simulink library "CommercialVehicleLibrary2G"  (R2021a)
settings: Solver=VariableStepAuto  StartTime=0.0  StopTime=10.0  RelTol=1e-3
values from neighbouring files (symbols this model uses):
  brake_input = [0   tmax ... (first row only)    [init_vehicle.m]    (also in run_Circle.m = [0  tmax; run_Coastdown.m = [0  2  tmax; run_DoubleLaneChangeDriver.m = [0   2  tmax; run_MaxAcc.m = [0  2  tmax)
  pose_t0 = [0 0 0 0]    [init_vehicle.m]    (also in run_Circle.m; run_Coastdown.m; run_DoubleLaneChangeDriver.m; run_MaxAcc.m)
  rdfname = 'TNO_FlatRoad.rdf'    [run_Circle.m]    (also in run_Coastdown.m; run_DoubleLaneChangeDriver.m; run_MaxAcc.m; run_Rollover.m)
  rdfname_inner = 'TNO_FlatRoad.rdf'    [run_Circle.m]    (also in run_Coastdown.m; run_DoubleLaneChangeDriver.m; run_MaxAcc.m; run_Rollover.m)
  steer_input = [0  tmax ... (first row only)    [init_vehicle.m]    (also in run_Circle.m = [0  2   10     13       tmax; run_Coastdown.m = [0 tmax; run_DoubleLaneChangeDriver.m = [0 tmax; run_MaxAcc.m = [0 tmax)
  throttle_input = [0         tmax ... (first row only)    [init_vehicle.m]    (also in run_Circle.m; run_Coastdown.m = [0        10         10.0001 tmax; run_DoubleLaneChangeDriver.m = [0        tmax; run_MaxAcc.m = [0        tmax)
  Vx = 0    [init_vehicle.m]    (also in run_Circle.m = Vx_kmh/3.6; run_Coastdown.m = Vx_kmh/3.6; run_DoubleLaneChangeDriver.m = Vx_kmh/3.6; run_MaxAcc.m)
  Vx_input = [0  tmax ... (first row only)    [init_vehicle.m]    (also in run_Circle.m; run_Coastdown.m = [0 tmax; run_DoubleLaneChangeDriver.m = [0 tmax; run_MaxAcc.m = [0 tmax)
undefined symbols (not defined in the file or in its folder): Drive, Floor, Fzstat, Fzstat1, Fzstat3, l, l_load1, l_load2, lbar, mass_load1, mass_load2, psi_semitrailer, rho, rim_Ixx, rim_Iyy, rim_mass, Steer, steer_path, tpfname, X, x_torsion, xcg, xcg1, xcg2, xcg_front, xcg_rear, xdrive1, xload1, xload2, xpos1, xref, xrev1, Xt0, Y, Yt0, Z
libraries: sm_lib x291, $bdroot x157, nesl_utility x143, vrlib x1
(part 12 of 12)

== system CommercialVehicleLibrary2G/Vehicles/Rigid Truck - 4 axles/Measurements ==
  Bus Creator2 : BusCreator  Inputs=3
  Bus Creator3 : BusCreator  Inputs=3
  Fcn4 : Fcn  Expr=u(3)
  PS-Simulink Converter{3..8,10..11} (8 alike) : nesl_utility/PS-Simulink Converter  PhysicalDomain=network_engine_domain  SubClassName=ps_output  LeftPortType=input  RightPortType=output  PseudoPeriodic=off  Frequencies=[]  Unit=inherit  AffineConversion=off
  Scope : Scope
  Scope1 : Scope
  Transform Sensor1 : sm_lib/Frames and Transforms/Transform Sensor  MeasurementFrame=NonRotatingFollower  SenseAngle=off  SenseAxis=off  SenseAngle1=off  SenseAngle2=off  SenseAngle3=off  SenseQ=off  SenseR=off  SenseOmegaX=on  SenseOmegaY=on  SenseOmegaZ=on  SenseOmega1=off  SenseOmega2=off  SenseOmega3=off  SenseQDot=off  SenseRDot=off  SenseAlphaX=on  SenseAlphaY=on  SenseAlphaZ=on  SenseAlpha1=off  SenseAlpha2=off  SenseAlpha3=off  SenseQDDot=off  SenseRDDot=off  SenseX=off  SenseY=off  SenseZ=off  SenseRad=off  SenseAzim=off  SenseDist=off  SenseInc=off  SenseXDot=on  SenseYDot=on  SenseZDot=off  SenseRadDot=off  SenseAzimDot=off  SenseDistDot=off  SenseIncDot=off  SenseXDDot=off  SenseYDDot=off  SenseZDDot=off  SenseRadDDot=off  SenseAzimDDot=off  SenseDistDDot=off  SenseIncDDot=off
  Transform Sensor2 : PMIOPort  Side=Left
  Transform Sensor3 : PMIOPort  Port=2  Side=Right
  Out1 : Outport
  Out2 : Outport  Port=2
  Out3 : Outport  Port=3
  wires:
  PS-Simulink Converter3/1 -> Bus Creator2/3
  PS-Simulink Converter5/1 -> Bus Creator2/1
  PS-Simulink Converter10/1 -> Scope1/1
  PS-Simulink Converter7/1 -> Bus Creator3/2
  Bus Creator2/1 -> Fcn4/1
  PS-Simulink Converter8/1 -> Bus Creator3/1
  Bus Creator3/1 -> Out2/1
  PS-Simulink Converter6/1 -> Bus Creator3/3
  PS-Simulink Converter4/1 -> Bus Creator2/2
  Fcn4/1 -> Out1/1
  PS-Simulink Converter11/1 -> Out3/1, Scope/1
  connections:
  PS-Simulink Converter11/LConn1 -- Transform Sensor1/RConn8
  PS-Simulink Converter7/LConn1 -- Transform Sensor1/RConn6
  Transform Sensor1/RConn2 -- PS-Simulink Converter5/LConn1
  PS-Simulink Converter6/LConn1 -- Transform Sensor1/RConn7
  PS-Simulink Converter3/LConn1 -- Transform Sensor1/RConn4
  Transform Sensor1/RConn1 -- Transform Sensor3/RConn1
  PS-Simulink Converter8/LConn1 -- Transform Sensor1/RConn5
  PS-Simulink Converter4/LConn1 -- Transform Sensor1/RConn3
  Transform Sensor1/RConn9 -- PS-Simulink Converter10/LConn1
  Transform Sensor1/LConn1 -- Transform Sensor2/RConn1

== system CommercialVehicleLibrary2G/Vehicles/Tractor/Cameras ==
  Front Camera Transform : sm_lib/Frames and Transforms/Rigid Transform  TranslationMethod=Cartesian  TranslationStandardOffset=0  TranslationLengthUnit=m  TranslationStandardAxis=+Z  TranslationCartesianOffset=[-10 0 6]  TranslationROffset=0  TranslationROffsetUnits=m  TranslationZOffset=0  TranslationZOffsetUnits=m  TranslationThetaOffset=0  TranslationThetaOffsetUnits=deg  RotationMethod=None  RotationAngleUnits=deg  RotationStandardAxis=+Y  RotationAngle=90  RotationArbitraryAxis=[0 0 1]  FollAlignAxisA=+X  BaseAlignAxisA=+Y  FollAlignAxisB=+Y  BaseAlignAxisB=+Z  RotationSequenceAxes=FollowerAxes  RotationSequence=XYX  RotationSequenceAngles=[0 0 0]  RotationSequenceAnglesUnits=deg  RotationMatrix=[1 0 0; 0 1 0; 0 0 1]
  Side Camera Transform : sm_lib/Frames and Transforms/Rigid Transform  TranslationMethod=Cartesian  TranslationStandardOffset=0  TranslationLengthUnit=m  TranslationStandardAxis=+Z  TranslationCartesianOffset=[5 3 3]  TranslationROffset=0  TranslationROffsetUnits=m  TranslationZOffset=0  TranslationZOffsetUnits=m  TranslationThetaOffset=0  TranslationThetaOffsetUnits=deg  RotationMethod=None  RotationAngleUnits=deg  RotationStandardAxis=+Z  RotationAngle=90  RotationArbitraryAxis=[0 0 1]  FollAlignAxisA=+X  BaseAlignAxisA=+Y  FollAlignAxisB=+Y  BaseAlignAxisB=+Z  RotationSequenceAxes=FollowerAxes  RotationSequence=XYX  RotationSequenceAngles=[0 0 0]  RotationSequenceAnglesUnits=deg  RotationMatrix=[1 0 0; 0 1 0; 0 0 1]
  Spherical Solid : sm_lib/Body Elements/Spherical Solid  GraphicAmbientColor=[0.15 0.15 0.15 1.0]  BasedOnType=Density  CenterOfMass=[0 0 0]  CenterOfMassUnits=m  GraphicDiffuseColor=[0.5 0.5 0.5]  Density=1000  DensityUnits=kg/m^3  DoExposeReferenceFrame=on  GraphicEmissiveColor=[0.0 0.0 0.0 1.0]  ExportEntireGeometry=off  SerializedExposedGeometries=<ExposedGeometries/>  SerializedFrames=<Frames/>  MarkerShape=Sphere  MarkerSize=10  GraphicType=FromGeometry  InertiaType=PointMass  Mass=1e-09  MassUnits=kg  MomentsOfInertia=[1 1 1]  MomentsOfInertiaUnits=kg*m^2  GraphicOpacity=0  ProductsOfInertia=[0 0 0]  ProductsOfInertiaUnits=kg*m^2  GraphicShininess=75  GraphicSpecularColor=[0.5 0.5 0.5 1.0]  SphereRadius=1e-09  SphereRadiusUnits=m  GraphicVisPropType=SimpleVisualProperties
  Spherical Solid1 : sm_lib/Body Elements/Spherical Solid  GraphicAmbientColor=[0.15 0.15 0.15 1.0]  BasedOnType=Density  CenterOfMass=[0 0 0]  CenterOfMassUnits=m  GraphicDiffuseColor=[0.5 0.5 0.5]  Density=1000  DensityUnits=kg/m^3  DoExposeReferenceFrame=on  GraphicEmissiveColor=[0.0 0.0 0.0 1.0]  ExportEntireGeometry=off  SerializedExposedGeometries=<ExposedGeometries/>  SerializedFrames=<Frames/>  MarkerShape=Sphere  MarkerSize=10  GraphicType=FromGeometry  InertiaType=PointMass  Mass=1e-09  MassUnits=kg  MomentsOfInertia=[1 1 1]  MomentsOfInertiaUnits=kg*m^2  GraphicOpacity=0  ProductsOfInertia=[0 0 0]  ProductsOfInertiaUnits=kg*m^2  GraphicShininess=75  GraphicSpecularColor=[0.5 0.5 0.5 1.0]  SphereRadius=1e-09  SphereRadiusUnits=m  GraphicVisPropType=SimpleVisualProperties
  " " : PMIOPort  Side=Left
  connections:
  Spherical Solid1/RConn1 -- Front Camera Transform/RConn1
  Spherical Solid/RConn1 -- Side Camera Transform/RConn1
  " "/RConn1 -- Front Camera Transform/LConn1 -- Side Camera Transform/LConn1

== system CommercialVehicleLibrary2G/Vehicles/Tractor/Measurements ==
  Bus Creator2 : BusCreator  Inputs=3
  Bus Creator3 : BusCreator  Inputs=3
  Fcn4 : Fcn  Expr=u(3)
  PS-Simulink Converter{3..8,10..11} (8 alike) : nesl_utility/PS-Simulink Converter  PhysicalDomain=network_engine_domain  SubClassName=ps_output  LeftPortType=input  RightPortType=output  PseudoPeriodic=off  Frequencies=[]  Unit=inherit  AffineConversion=off
  Scope : Scope
  Scope1 : Scope
  Transform Sensor1 : sm_lib/Frames and Transforms/Transform Sensor  MeasurementFrame=NonRotatingFollower  SenseAngle=off  SenseAxis=off  SenseAngle1=off  SenseAngle2=off  SenseAngle3=off  SenseQ=off  SenseR=off  SenseOmegaX=on  SenseOmegaY=on  SenseOmegaZ=on  SenseOmega1=off  SenseOmega2=off  SenseOmega3=off  SenseQDot=off  SenseRDot=off  SenseAlphaX=on  SenseAlphaY=on  SenseAlphaZ=on  SenseAlpha1=off  SenseAlpha2=off  SenseAlpha3=off  SenseQDDot=off  SenseRDDot=off  SenseX=off  SenseY=off  SenseZ=off  SenseRad=off  SenseAzim=off  SenseDist=off  SenseInc=off  SenseXDot=on  SenseYDot=on  SenseZDot=off  SenseRadDot=off  SenseAzimDot=off  SenseDistDot=off  SenseIncDot=off  SenseXDDot=off  SenseYDDot=off  SenseZDDot=off  SenseRadDDot=off  SenseAzimDDot=off  SenseDistDDot=off  SenseIncDDot=off
  Transform Sensor2 : PMIOPort  Side=Left
  Transform Sensor3 : PMIOPort  Port=2  Side=Right
  Out1 : Outport
  Out2 : Outport  Port=2
  Out3 : Outport  Port=3
  wires:
  PS-Simulink Converter11/1 -> Scope/1, Out3/1
  Fcn4/1 -> Out1/1
  PS-Simulink Converter4/1 -> Bus Creator2/2
  PS-Simulink Converter6/1 -> Bus Creator3/3
  Bus Creator3/1 -> Out2/1
  PS-Simulink Converter8/1 -> Bus Creator3/1
  Bus Creator2/1 -> Fcn4/1
  PS-Simulink Converter7/1 -> Bus Creator3/2
  PS-Simulink Converter10/1 -> Scope1/1
  PS-Simulink Converter5/1 -> Bus Creator2/1
  PS-Simulink Converter3/1 -> Bus Creator2/3
  connections:
  Transform Sensor1/LConn1 -- Transform Sensor2/RConn1
  Transform Sensor1/RConn9 -- PS-Simulink Converter10/LConn1
  PS-Simulink Converter4/LConn1 -- Transform Sensor1/RConn3
  PS-Simulink Converter8/LConn1 -- Transform Sensor1/RConn5
  Transform Sensor1/RConn1 -- Transform Sensor3/RConn1
  PS-Simulink Converter3/LConn1 -- Transform Sensor1/RConn4
  PS-Simulink Converter6/LConn1 -- Transform Sensor1/RConn7
  Transform Sensor1/RConn2 -- PS-Simulink Converter5/LConn1
  PS-Simulink Converter7/LConn1 -- Transform Sensor1/RConn6
  PS-Simulink Converter11/LConn1 -- Transform Sensor1/RConn8

== system CommercialVehicleLibrary2G/Combinations/LZV_B/To_workspace_semitrailer1/Subsystem ==
  In1 : Inport
  Bus Selector24 : BusSelector  OutputSignals=axle1.Tire_L.Fx,axle1.Tire_R.Fx,axle2.Tire_L.Fx,axle2.Tire_R.Fx,axle3.Tire_L.Fx,axle3.Tire_R.Fx
  Mux : Mux  Inputs=6
  Out1 : Outport
  wires:
  Bus Selector24/4 -> Mux/4  "<Fx>"
  Bus Selector24/3 -> Mux/3  "<Fx>"
  Bus Selector24/2 -> Mux/2  "<Fx>"
  Bus Selector24/1 -> Mux/1  "<Fx>"
  Mux/1 -> Out1/1
  In1/1 -> Bus Selector24/1
  Bus Selector24/5 -> Mux/5  "<Fx>"
  Bus Selector24/6 -> Mux/6  "<Fx>"

== system CommercialVehicleLibrary2G/Combinations/LZV_B/To_workspace_semitrailer1/Subsystem1 ==
  In1 : Inport
  Bus Selector24 : BusSelector  OutputSignals=axle1.Tire_L.Fy,axle1.Tire_R.Fy,axle2.Tire_L.Fy,axle2.Tire_R.Fy,axle3.Tire_L.Fy,axle3.Tire_R.Fy
  Mux : Mux  Inputs=6
  Out1 : Outport
  wires:
  Mux/1 -> Out1/1
  In1/1 -> Bus Selector24/1
  Bus Selector24/1 -> Mux/1  "<Fy>"
  Bus Selector24/2 -> Mux/2  "<Fy>"
  Bus Selector24/3 -> Mux/3  "<Fy>"
  Bus Selector24/4 -> Mux/4  "<Fy>"
  Bus Selector24/5 -> Mux/5  "<Fy>"
  Bus Selector24/6 -> Mux/6  "<Fy>"

== system CommercialVehicleLibrary2G/Combinations/LZV_B/To_workspace_semitrailer1/Subsystem2 ==
  In1 : Inport
  Bus Selector24 : BusSelector  OutputSignals=axle1.Tire_L.Fz,axle1.Tire_R.Fz,axle2.Tire_L.Fz,axle2.Tire_R.Fz,axle3.Tire_L.Fz,axle3.Tire_R.Fz
  Mux : Mux  Inputs=6
  Out1 : Outport
  wires:
  Mux/1 -> Out1/1
  In1/1 -> Bus Selector24/1
  Bus Selector24/1 -> Mux/1  "<Fz>"
  Bus Selector24/2 -> Mux/2  "<Fz>"
  Bus Selector24/3 -> Mux/3  "<Fz>"
  Bus Selector24/4 -> Mux/4  "<Fz>"
  Bus Selector24/5 -> Mux/5  "<Fz>"
  Bus Selector24/6 -> Mux/6  "<Fz>"

== system CommercialVehicleLibrary2G/Combinations/LZV_B/To_workspace_semitrailer1/Subsystem3 ==
  In1 : Inport
  Bus Selector6 : BusSelector  OutputSignals=axle1.Omega1,axle1.Omega2,axle2.Omega1,axle2.Omega2,axle3.Omega1,axle3.Omega2
  Mux : Mux  Inputs=6
  Out1 : Outport
  wires:
  In1/1 -> Bus Selector6/1
  Mux/1 -> Out1/1
  Bus Selector6/1 -> Mux/1  "<Omega1>"
  Bus Selector6/2 -> Mux/2  "<Omega2>"
  Bus Selector6/3 -> Mux/3  "<Omega1>"
  Bus Selector6/4 -> Mux/4  "<Omega2>"
  Bus Selector6/5 -> Mux/5  "<Omega1>"
  Bus Selector6/6 -> Mux/6  "<Omega2>"

== system CommercialVehicleLibrary2G/Combinations/LZV_B/To_workspace_semitrailer2/Subsystem ==
  In1 : Inport
  Bus Selector24 : BusSelector  OutputSignals=axle1.Tire_L.Fx,axle1.Tire_R.Fx,axle2.Tire_L.Fx,axle2.Tire_R.Fx,axle3.Tire_L.Fx,axle3.Tire_R.Fx
  Mux : Mux  Inputs=6
  Out1 : Outport
  wires:
  Bus Selector24/6 -> Mux/6  "<Fx>"
  Bus Selector24/5 -> Mux/5  "<Fx>"
  In1/1 -> Bus Selector24/1
  Mux/1 -> Out1/1
  Bus Selector24/1 -> Mux/1  "<Fx>"
  Bus Selector24/2 -> Mux/2  "<Fx>"
  Bus Selector24/3 -> Mux/3  "<Fx>"
  Bus Selector24/4 -> Mux/4  "<Fx>"

== system CommercialVehicleLibrary2G/Combinations/LZV_B/To_workspace_semitrailer2/Subsystem1 ==
  In1 : Inport
  Bus Selector24 : BusSelector  OutputSignals=axle1.Tire_L.Fy,axle1.Tire_R.Fy,axle2.Tire_L.Fy,axle2.Tire_R.Fy,axle3.Tire_L.Fy,axle3.Tire_R.Fy
  Mux : Mux  Inputs=6
  Out1 : Outport
  wires:
  Bus Selector24/6 -> Mux/6  "<Fy>"
  Bus Selector24/5 -> Mux/5  "<Fy>"
  Bus Selector24/4 -> Mux/4  "<Fy>"
  Bus Selector24/3 -> Mux/3  "<Fy>"
  Bus Selector24/2 -> Mux/2  "<Fy>"
  Bus Selector24/1 -> Mux/1  "<Fy>"
  In1/1 -> Bus Selector24/1
  Mux/1 -> Out1/1

== system CommercialVehicleLibrary2G/Combinations/LZV_B/To_workspace_semitrailer2/Subsystem2 ==
  In1 : Inport
  Bus Selector24 : BusSelector  OutputSignals=axle1.Tire_L.Fz,axle1.Tire_R.Fz,axle2.Tire_L.Fz,axle2.Tire_R.Fz,axle3.Tire_L.Fz,axle3.Tire_R.Fz
  Mux : Mux  Inputs=6
  Out1 : Outport
  wires:
  Bus Selector24/6 -> Mux/6  "<Fz>"
  Bus Selector24/5 -> Mux/5  "<Fz>"
  Bus Selector24/4 -> Mux/4  "<Fz>"
  Bus Selector24/3 -> Mux/3  "<Fz>"
  Bus Selector24/2 -> Mux/2  "<Fz>"
  Bus Selector24/1 -> Mux/1  "<Fz>"
  In1/1 -> Bus Selector24/1
  Mux/1 -> Out1/1

== system CommercialVehicleLibrary2G/Combinations/LZV_B/To_workspace_semitrailer2/Subsystem3 ==
  In1 : Inport
  Bus Selector6 : BusSelector  OutputSignals=axle1.Omega1,axle1.Omega2,axle2.Omega1,axle2.Omega2,axle3.Omega1,axle3.Omega2
  Mux : Mux  Inputs=6
  Out1 : Outport
  wires:
  Bus Selector6/6 -> Mux/6  "<Omega2>"
  Bus Selector6/5 -> Mux/5  "<Omega1>"
  Bus Selector6/4 -> Mux/4  "<Omega2>"
  Bus Selector6/3 -> Mux/3  "<Omega1>"
  Bus Selector6/2 -> Mux/2  "<Omega2>"
  Bus Selector6/1 -> Mux/1  "<Omega1>"
  Mux/1 -> Out1/1
  In1/1 -> Bus Selector6/1

== system CommercialVehicleLibrary2G/Combinations/LZV_E/To_workspace_drawbar_trailer_2axle 2/Subsystem ==
  In1 : Inport
  Bus Selector24 : BusSelector  OutputSignals=axle1.Tire_L.Fx,axle1.Tire_R.Fx,axle2.Tire_L.Fx,axle2.Tire_R.Fx
  Mux : Mux
  Out1 : Outport
  wires:
  Bus Selector24/4 -> Mux/4  "<Fx>"
  Bus Selector24/3 -> Mux/3  "<Fx>"
  Bus Selector24/2 -> Mux/2  "<Fx>"
  Bus Selector24/1 -> Mux/1  "<Fx>"
  Mux/1 -> Out1/1
  In1/1 -> Bus Selector24/1

== system CommercialVehicleLibrary2G/Combinations/LZV_E/To_workspace_drawbar_trailer_2axle 2/Subsystem1 ==
  In1 : Inport
  Bus Selector24 : BusSelector  OutputSignals=axle1.Tire_L.Fy,axle1.Tire_R.Fy,axle2.Tire_L.Fy,axle2.Tire_R.Fy
  Mux : Mux
  Out1 : Outport
  wires:
  Mux/1 -> Out1/1
  In1/1 -> Bus Selector24/1
  Bus Selector24/1 -> Mux/1  "<Fy>"
  Bus Selector24/2 -> Mux/2  "<Fy>"
  Bus Selector24/3 -> Mux/3  "<Fy>"
  Bus Selector24/4 -> Mux/4  "<Fy>"

== system CommercialVehicleLibrary2G/Combinations/LZV_E/To_workspace_drawbar_trailer_2axle 2/Subsystem2 ==
  In1 : Inport
  Bus Selector24 : BusSelector  OutputSignals=axle1.Tire_L.Fz,axle1.Tire_R.Fz,axle2.Tire_L.Fz,axle2.Tire_R.Fz
  Mux : Mux
  Out1 : Outport
  wires:
  Mux/1 -> Out1/1
  In1/1 -> Bus Selector24/1
  Bus Selector24/1 -> Mux/1  "<Fz>"
  Bus Selector24/2 -> Mux/2  "<Fz>"
  Bus Selector24/3 -> Mux/3  "<Fz>"
  Bus Selector24/4 -> Mux/4  "<Fz>"

== system CommercialVehicleLibrary2G/Combinations/LZV_E/To_workspace_drawbar_trailer_2axle 2/Subsystem3 ==
  In1 : Inport
  Bus Selector6 : BusSelector  OutputSignals=axle1.Omega1,axle1.Omega2,axle2.Omega1,axle2.Omega2
  Mux : Mux
  Out1 : Outport
  wires:
  In1/1 -> Bus Selector6/1
  Mux/1 -> Out1/1
  Bus Selector6/1 -> Mux/1  "<Omega1>"
  Bus Selector6/2 -> Mux/2  "<Omega2>"
  Bus Selector6/3 -> Mux/3  "<Omega1>"
  Bus Selector6/4 -> Mux/4  "<Omega2>"

== matlab function CommercialVehicleLibrary2G/Assemblies/Driver/PreviewSteering/Embedded MATLAB Function ==
  data: line input; dist output; point input; npoints input; idx1 input; pos output; idx2 output
function [dist,pos,idx2] = dist2line(line,point,npoints,idx1)
% This block supports the Embedded MATLAB subset.
% See the help menu for details. 

a  =[0 0 0]';
b  =[0 0 0]';
c  =[0 0 0]';
pos=[0 0 0]';
mdist=[0];

idx=idx1;

if idx < 0
  idx_min = 1;
  idx_max = length(line);
else
  idx_min = max(1,idx-npoints);
  idx_max = min(length(line),idx+npoints);
end

idx_min_dist = 0;
min_dist     = 1e8;

for i=idx_min:idx_max
  mdist = norm( line(:,i) - point );
  if mdist < min_dist
    idx = i;
    min_dist = mdist;
    pos = line(:,i);
  end
end

idx=max(idx,2);
idx=min(idx,length(line)-1);

for i=idx-1:idx
  a = line(:,i+1) - line(:,i);
  b = point - line(:,i);
  
  alpha = dot(a,b)/dot(a,a);
  dist  = norm(b - alpha*a);
  
  if alpha > 0 && alpha < 1 && dist < min_dist
    min_dist= dist;
    pos = line(:,i)+alpha*a;
    idx = i;
    c=cross(a,b);
    dist_sgn = sign(c(3));
  end
end

a = line(:,idx+1) - line(:,idx);
b = point - pos;
c = cross(a,b);
dist_sgn = sign(c(3));

dist = min_dist*dist_sgn;
idx2=idx;
